simulink model "Model_Testing"  (R2022a)
settings: Solver=VariableStepAuto  StartTime=0.0  StopTime=10.0  RelTol=1e-3
undefined symbols (not defined in the file): m, r
settings Model: Creator=Bastien C  LastModifiedBy=Bastien C

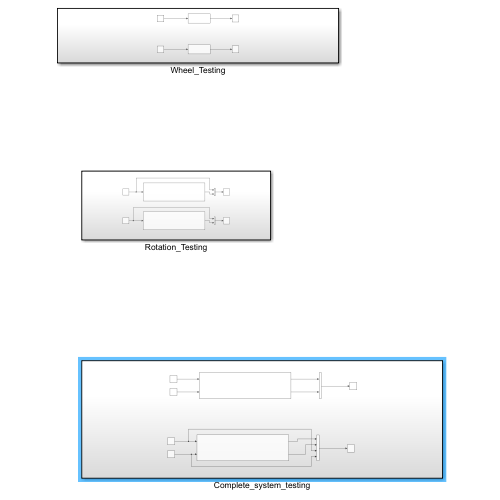
[thumbnail: Simulink's stored preview of the top-level diagram]
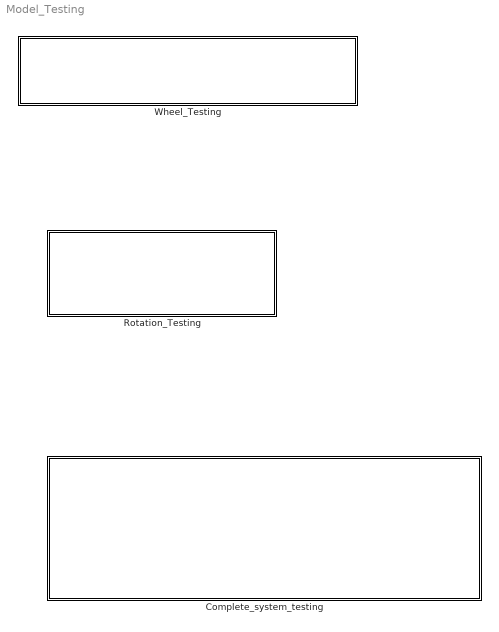
== system Model_Testing ==
  Complete_system_testing : Subsystem
  Rotation_Testing : Subsystem
  Wheel_Testing : Subsystem

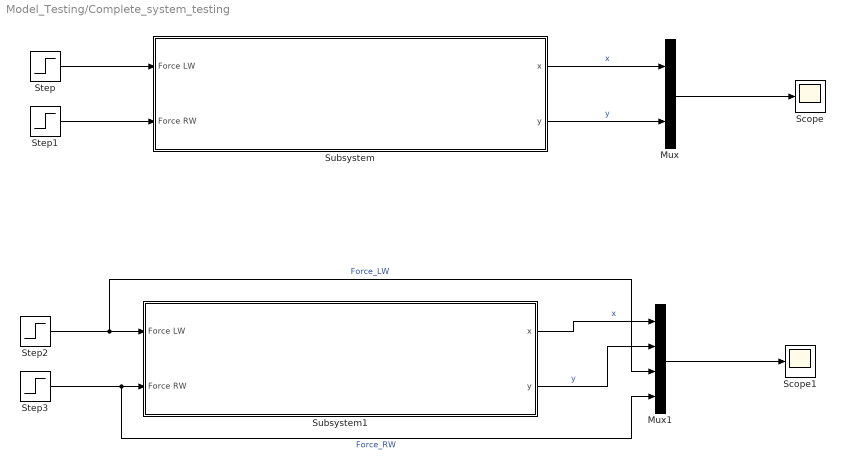
== system Model_Testing/Complete_system_testing ==
  Mux : Mux  Inputs=2
  Mux1 : Mux
  Scope : Scope
  Scope1 : Scope
  Step : Step  SampleTime=0
  Step1 : Step  SampleTime=0
  Step2 : Step  Before=0.5  SampleTime=0
  Step3 : Step  Before=0.5  After=-1  SampleTime=0
  Subsystem : Subsystem
  Subsystem1 : Subsystem
  wires:
  Subsystem/2(y) -> Mux/2  "y"
  Subsystem/1(x) -> Mux/1  "x"
  Step/1 -> Subsystem/1(Force LW)
  Step1/1 -> Subsystem/2(Force RW)
  Mux/1 -> Scope/1
  Mux1/1 -> Scope1/1
  Step3/1 -> Mux1/4, Subsystem1/2(Force RW)  "Force_RW"
  Step2/1 -> Mux1/3, Subsystem1/1(Force LW)  "Force_LW"
  Subsystem1/1(x) -> Mux1/1  "x"
  Subsystem1/2(y) -> Mux1/2  "y"

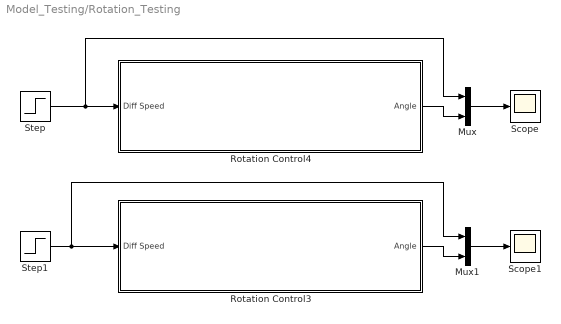
== system Model_Testing/Rotation_Testing ==
  Mux : Mux  Inputs=2
  Mux1 : Mux  Inputs=2
  Rotation Control3 : Subsystem
  Rotation Control4 : Subsystem
  Scope : Scope
  Scope1 : Scope
  Step : Step  SampleTime=0
  Step1 : Step  Time=2  Before=1  After=-1  SampleTime=0
  wires:
  Step/1 -> Mux/1, Rotation Control4/1(Diff Speed)
  Step1/1 -> Mux1/1, Rotation Control3/1(Diff Speed)
  Rotation Control4/1(Angle) -> Mux/2
  Rotation Control3/1(Angle) -> Mux1/2
  Mux/1 -> Scope/1
  Mux1/1 -> Scope1/1

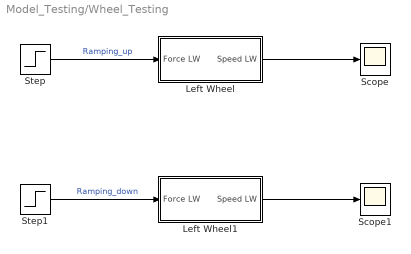
== system Model_Testing/Wheel_Testing ==
  Left Wheel : Subsystem
  Left Wheel1 : Subsystem
  Scope : Scope
  Scope1 : Scope
  Step : Step  SampleTime=0
  Step1 : Step  Time=3  Before=1  After=0  SampleTime=0
  wires:
  Left Wheel1/1(Speed LW) -> Scope1/1
  Step/1 -> Left Wheel/1(Force LW)  "Ramping_up"
  Step1/1 -> Left Wheel1/1(Force LW)  "Ramping_down"
  Left Wheel/1(Speed LW) -> Scope/1

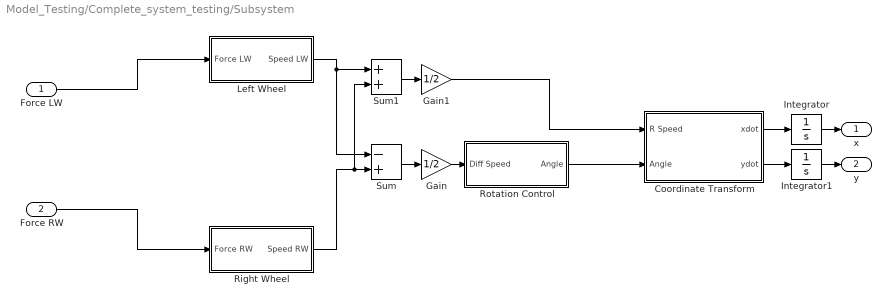
== system Model_Testing/Complete_system_testing/Subsystem ==
  Force LW : Inport
  Force RW : Inport  Port=2
  Coordinate Transform : Subsystem
  Gain : Gain  Gain=1/2
  Gain1 : Gain  Gain=1/2
  Integrator : Integrator
  Integrator1 : Integrator
  Left Wheel : Subsystem
  Right Wheel : Subsystem
  Rotation Control : Subsystem
  Sum : Sum  Inputs=-+
  Sum1 : Sum
  x : Outport
  y : Outport  Port=2
  wires:
  Left Wheel/1(Speed LW) -> Sum1/1, Sum/1
  Gain/1 -> Rotation Control/1(Diff Speed)
  Gain1/1 -> Coordinate Transform/1(R Speed)
  Sum/1 -> Gain/1
  Force LW/1 -> Left Wheel/1(Force LW)
  Coordinate Transform/1(xdot) -> Integrator/1
  Rotation Control/1(Angle) -> Coordinate Transform/2(Angle)
  Right Wheel/1(Speed RW) -> Sum1/2, Sum/2
  Sum1/1 -> Gain1/1
  Force RW/1 -> Right Wheel/1(Force RW)
  Coordinate Transform/2(ydot) -> Integrator1/1
  Integrator/1 -> x/1
  Integrator1/1 -> y/1

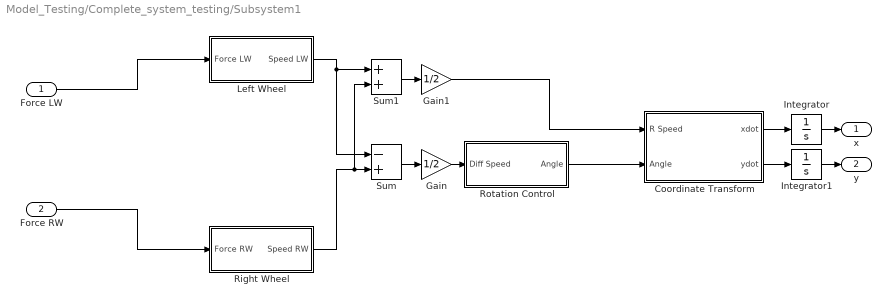
== system Model_Testing/Complete_system_testing/Subsystem1 ==
  Force LW : Inport
  Force RW : Inport  Port=2
  Coordinate Transform : Subsystem
  Gain : Gain  Gain=1/2
  Gain1 : Gain  Gain=1/2
  Integrator : Integrator
  Integrator1 : Integrator
  Left Wheel : Subsystem
  Right Wheel : Subsystem
  Rotation Control : Subsystem
  Sum : Sum  Inputs=-+
  Sum1 : Sum
  x : Outport
  y : Outport  Port=2
  wires:
  Integrator1/1 -> y/1
  Integrator/1 -> x/1
  Coordinate Transform/2(ydot) -> Integrator1/1
  Force RW/1 -> Right Wheel/1(Force RW)
  Sum1/1 -> Gain1/1
  Right Wheel/1(Speed RW) -> Sum/2, Sum1/2
  Rotation Control/1(Angle) -> Coordinate Transform/2(Angle)
  Coordinate Transform/1(xdot) -> Integrator/1
  Force LW/1 -> Left Wheel/1(Force LW)
  Sum/1 -> Gain/1
  Gain1/1 -> Coordinate Transform/1(R Speed)
  Gain/1 -> Rotation Control/1(Diff Speed)
  Left Wheel/1(Speed LW) -> Sum/1, Sum1/1

== system Model_Testing/Rotation_Testing/Rotation Control3 ==
  Diff Speed : Inport
  Gain : Gain  Gain=1/r
  Integrator : Integrator
  Angle : Outport
  wires:
  Gain/1 -> Integrator/1
  Integrator/1 -> Angle/1
  Diff Speed/1 -> Gain/1

== system Model_Testing/Rotation_Testing/Rotation Control4 ==
  Diff Speed : Inport
  Gain : Gain  Gain=1/r
  Integrator : Integrator
  Angle : Outport
  wires:
  Diff Speed/1 -> Gain/1
  Integrator/1 -> Angle/1
  Gain/1 -> Integrator/1

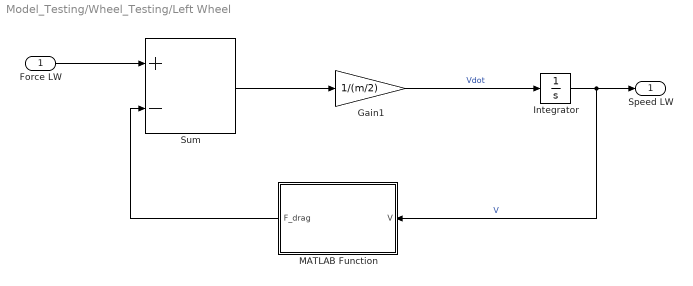
== system Model_Testing/Wheel_Testing/Left Wheel ==
  Force LW : Inport
  Gain1 : Gain  Gain=1/(m/2)
  Integrator : Integrator
  MATLAB Function : MATLAB Function  TreatAsAtomicUnit=on
  Sum : Sum  Inputs=+-
  Speed LW : Outport
  wires:
  Force LW/1 -> Sum/1
  Sum/1 -> Gain1/1
  Integrator/1 -> Speed LW/1, MATLAB Function/1(V)  "V"
  Gain1/1 -> Integrator/1  "Vdot"
  MATLAB Function/1(F_drag) -> Sum/2

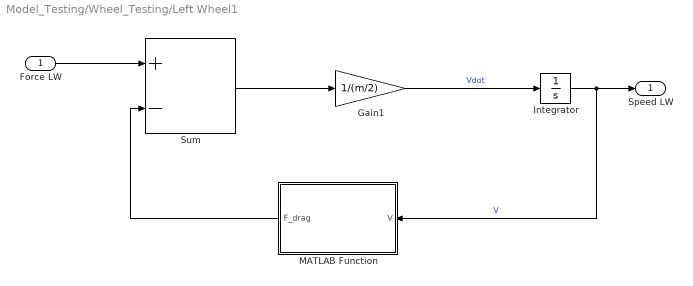
== system Model_Testing/Wheel_Testing/Left Wheel1 ==
  Force LW : Inport
  Gain1 : Gain  Gain=1/(m/2)
  Integrator : Integrator
  MATLAB Function : MATLAB Function  TreatAsAtomicUnit=on
  Sum : Sum  Inputs=+-
  Speed LW : Outport
  wires:
  MATLAB Function/1(F_drag) -> Sum/2
  Gain1/1 -> Integrator/1  "Vdot"
  Integrator/1 -> MATLAB Function/1(V), Speed LW/1  "V"
  Sum/1 -> Gain1/1
  Force LW/1 -> Sum/1

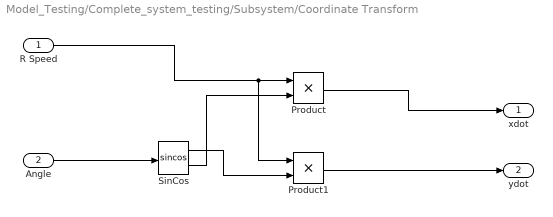
== system Model_Testing/Complete_system_testing/Subsystem/Coordinate Transform ==
  R Speed : Inport
  Angle : Inport  Port=2
  Product : Product
  Product1 : Product
  SinCos : Trigonometry  Operator=sincos
  xdot : Outport
  ydot : Outport  Port=2
  wires:
  R Speed/1 -> Product1/1, Product/1
  Product/1 -> xdot/1
  Product1/1 -> ydot/1
  Angle/1 -> SinCos/1
  SinCos/1 -> Product1/2
  SinCos/2 -> Product/2

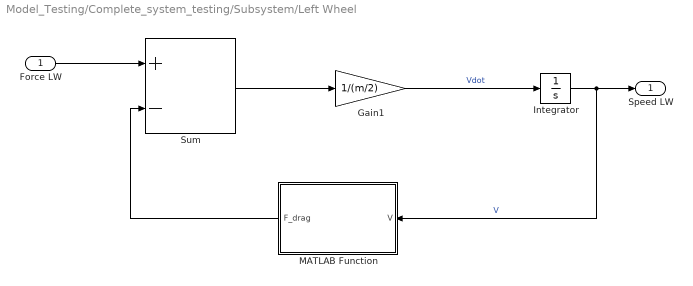
== system Model_Testing/Complete_system_testing/Subsystem/Left Wheel ==
  Force LW : Inport
  Gain1 : Gain  Gain=1/(m/2)
  Integrator : Integrator
  MATLAB Function : MATLAB Function  TreatAsAtomicUnit=on
  Sum : Sum  Inputs=+-
  Speed LW : Outport
  wires:
  Force LW/1 -> Sum/1
  Sum/1 -> Gain1/1
  Integrator/1 -> Speed LW/1, MATLAB Function/1(V)  "V"
  Gain1/1 -> Integrator/1  "Vdot"
  MATLAB Function/1(F_drag) -> Sum/2

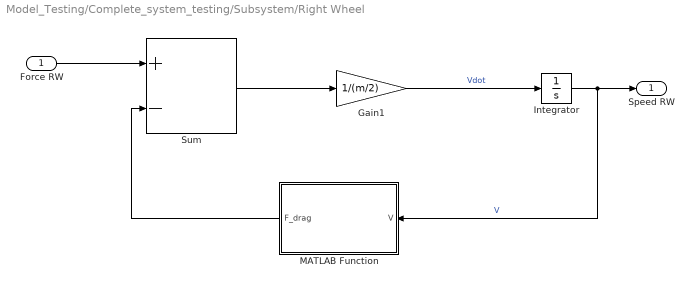
== system Model_Testing/Complete_system_testing/Subsystem/Right Wheel ==
  Force RW : Inport
  Gain1 : Gain  Gain=1/(m/2)
  Integrator : Integrator
  MATLAB Function : MATLAB Function  TreatAsAtomicUnit=on
  Sum : Sum  Inputs=+-
  Speed RW : Outport
  wires:
  Integrator/1 -> Speed RW/1, MATLAB Function/1(V)  "V"
  Force RW/1 -> Sum/1
  Sum/1 -> Gain1/1
  Gain1/1 -> Integrator/1  "Vdot"
  MATLAB Function/1(F_drag) -> Sum/2

== system Model_Testing/Complete_system_testing/Subsystem/Rotation Control ==
  Diff Speed : Inport
  Gain : Gain  Gain=1/r
  Integrator : Integrator
  Angle : Outport
  wires:
  Diff Speed/1 -> Gain/1
  Integrator/1 -> Angle/1
  Gain/1 -> Integrator/1

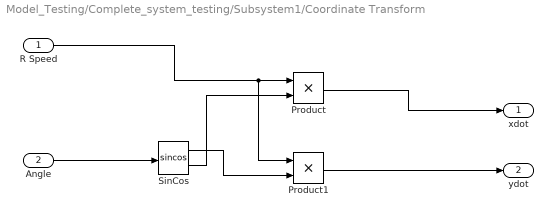
== system Model_Testing/Complete_system_testing/Subsystem1/Coordinate Transform ==
  R Speed : Inport
  Angle : Inport  Port=2
  Product : Product
  Product1 : Product
  SinCos : Trigonometry  Operator=sincos
  xdot : Outport
  ydot : Outport  Port=2
  wires:
  SinCos/2 -> Product/2
  SinCos/1 -> Product1/2
  Angle/1 -> SinCos/1
  Product1/1 -> ydot/1
  Product/1 -> xdot/1
  R Speed/1 -> Product/1, Product1/1

== system Model_Testing/Complete_system_testing/Subsystem1/Left Wheel ==
  Force LW : Inport
  Gain1 : Gain  Gain=1/(m/2)
  Integrator : Integrator
  MATLAB Function : MATLAB Function  TreatAsAtomicUnit=on
  Sum : Sum  Inputs=+-
  Speed LW : Outport
  wires:
  MATLAB Function/1(F_drag) -> Sum/2
  Gain1/1 -> Integrator/1  "Vdot"
  Integrator/1 -> MATLAB Function/1(V), Speed LW/1  "V"
  Sum/1 -> Gain1/1
  Force LW/1 -> Sum/1

== system Model_Testing/Complete_system_testing/Subsystem1/Right Wheel ==
  Force RW : Inport
  Gain1 : Gain  Gain=1/(m/2)
  Integrator : Integrator
  MATLAB Function : MATLAB Function  TreatAsAtomicUnit=on
  Sum : Sum  Inputs=+-
  Speed RW : Outport
  wires:
  MATLAB Function/1(F_drag) -> Sum/2
  Gain1/1 -> Integrator/1  "Vdot"
  Sum/1 -> Gain1/1
  Force RW/1 -> Sum/1
  Integrator/1 -> MATLAB Function/1(V), Speed RW/1  "V"

== system Model_Testing/Complete_system_testing/Subsystem1/Rotation Control ==
  Diff Speed : Inport
  Gain : Gain  Gain=1/r
  Integrator : Integrator
  Angle : Outport
  wires:
  Gain/1 -> Integrator/1
  Integrator/1 -> Angle/1
  Diff Speed/1 -> Gain/1

== matlab function Model_Testing/Wheel_Testing/Left Wheel/MATLAB Function ==
  data: V input; F_drag output; k_drag parameter
function F_drag = get_Fdrag(V, k_drag)

F_drag = k_drag * V * abs(V);

== matlab function Model_Testing/Complete_system_testing/Subsystem/Left Wheel/MATLAB Function ==
  data: V input; F_drag output; k_drag parameter
function F_drag = get_Fdrag(V, k_drag)

F_drag = k_drag * V * abs(V);

== matlab function Model_Testing/Complete_system_testing/Subsystem/Right Wheel/MATLAB Function ==
  data: V input; F_drag output; k_drag parameter
function F_drag = get_Fdrag(V, k_drag)

F_drag = k_drag * V * abs(V);

== matlab function Model_Testing/Complete_system_testing/Subsystem1/Left Wheel/MATLAB Function ==
  data: V input; F_drag output; k_drag parameter
function F_drag = get_Fdrag(V, k_drag)

F_drag = k_drag * V * abs(V);

== matlab function Model_Testing/Complete_system_testing/Subsystem1/Right Wheel/MATLAB Function ==
  data: V input; F_drag output; k_drag parameter
function F_drag = get_Fdrag(V, k_drag)

F_drag = k_drag * V * abs(V);

== matlab function Model_Testing/Wheel_Testing/Left Wheel1/MATLAB Function ==
  data: V input; F_drag output; k_drag parameter
function F_drag = get_Fdrag(V, k_drag)

F_drag = k_drag * V * abs(V);
